simulink subsystem "atm"  (R2022b)
settings: Solver=VariableStepAuto  StartTime=0.0  StopTime=10.0  RelTol=1e-3
libraries: dspsigops x3
settings Model: Creator=padlewsk  LastModifiedBy=padlewsk

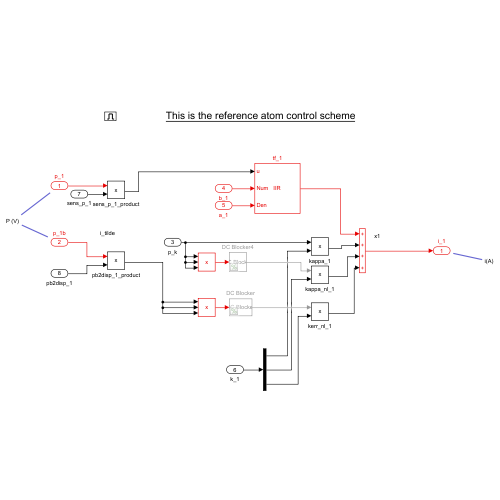
[thumbnail: Simulink's stored preview of the top-level diagram]
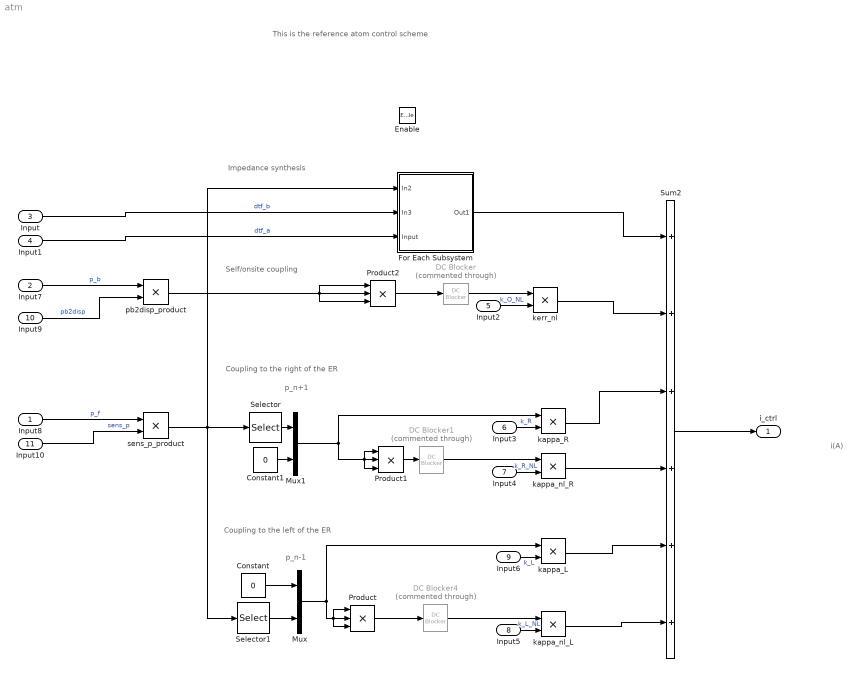
== system atm ==
  note: Impedance synthesis
  note: Coupling to the left of the ER
  note: Coupling to the right of the ER
  note: p_n-1
  note: This is the reference atom control scheme
  note: i(A)
  note: p_n+1
  note: Self/onsite coupling
  Input8 : Inport
  Input7 : Inport  Port=2
  Input : Inport  Port=3
  Input1 : Inport  Port=4
  Input2 : Inport  Port=5
  Input3 : Inport  Port=6
  Input4 : Inport  Port=7
  Input5 : Inport  Port=8
  Input6 : Inport  Port=9
  Input9 : Inport  Port=10
  Input10 : Inport  Port=11
  Enable : EnablePort
  Constant : Constant  Value=0
  Constant1 : Constant  Value=0
  DC Blocker : dspsigops/DC Blocker  Commented=through  Algorithm=FIR  NormalizedBandwidth=0.001  Length=50  Order=6  SimulateUsing=Code generation
      settings: LibrarySourceBlock=dsphdlsupportsigops/DC Blocker
  DC Blocker1 : dspsigops/DC Blocker  Commented=through  Algorithm=FIR  NormalizedBandwidth=0.001  Length=50  Order=6  SimulateUsing=Code generation
      settings: LibrarySourceBlock=dsphdlsupportsigops/DC Blocker
  DC Blocker4 : dspsigops/DC Blocker  Commented=through  Algorithm=FIR  NormalizedBandwidth=0.001  Length=50  Order=6  SimulateUsing=Code generation
      settings: LibrarySourceBlock=dsphdlsupportsigops/DC Blocker
  For Each Subsystem : Subsystem  TreatAsAtomicUnit=on
      settings: MinAlgLoopOccurrences=on  RTWSystemCode=Nonreusable function
  Mux : Mux  Inputs=2
  Mux1 : Mux  Inputs=2
  Product : Product  Inputs=3
  Product1 : Product  Inputs=3
  Product2 : Product  Inputs=3
  Selector : Selector  InputPortWidth=16  IndexOptions=Index vector (dialog)  Indices=[2:16]  OutputSizes=1
  Selector1 : Selector  InputPortWidth=16  IndexOptions=Index vector (dialog)  Indices=[1:15]  OutputSizes=1
  Sum2 : Sum  Inputs=++++++
  kappa_L : Product
  kappa_R : Product
  kappa_nl_L : Product
  kappa_nl_R : Product
  kerr_nl : Product
  pb2disp_product : Product
  sens_p_product : Product
  i_ctrl : Outport
  wires:
  Sum2/1 -> i_ctrl/1
  pb2disp_product/1 -> Product2/2, Product2/1, Product2/3
  Product/1 -> DC Blocker4/1
  DC Blocker4/1 -> kappa_nl_L/1
  DC Blocker/1 -> kerr_nl/1
  Product2/1 -> DC Blocker/1
  Product1/1 -> DC Blocker1/1
  DC Blocker1/1 -> kappa_nl_R/1
  kerr_nl/1 -> Sum2/2
  Constant/1 -> Mux/1
  Constant1/1 -> Mux1/2
  sens_p_product/1 -> Selector/1, Selector1/1, For Each Subsystem/1(In2)
  Mux1/1 -> Product1/2, Product1/1, Product1/3, kappa_R/1
  Mux/1 -> Product/2, Product/1, Product/3, kappa_L/1
  Selector/1 -> Mux1/1
  Selector1/1 -> Mux/2
  kappa_R/1 -> Sum2/3
  kappa_nl_R/1 -> Sum2/4
  kappa_L/1 -> Sum2/5
  kappa_nl_L/1 -> Sum2/6
  Input/1 -> For Each Subsystem/2(In3)  "dtf_b"
  Input1/1 -> For Each Subsystem/3(Input)  "dtf_a"
  Input4/1 -> kappa_nl_R/2  "k_R_NL"
  Input2/1 -> kerr_nl/2  "k_O_NL"
  Input3/1 -> kappa_R/2  "k_R"
  Input5/1 -> kappa_nl_L/2  "k_L_NL"
  Input6/1 -> kappa_L/2  "k_L"
  Input7/1 -> pb2disp_product/1  "p_b"
  Input8/1 -> sens_p_product/1  "p_f"
  Input9/1 -> pb2disp_product/2  "pb2disp"
  Input10/1 -> sens_p_product/2  "sens_p"
  For Each Subsystem/1(Out1) -> Sum2/1

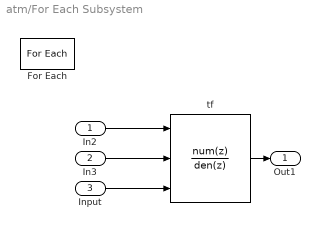
== system atm/For Each Subsystem ==
  In2 : Inport  Partition=on  PartitionDimension=1  PartitionWidth=1  PartitionOffset=0
  In3 : Inport  Port=2  Partition=on  PartitionDimension=1  PartitionWidth=1  PartitionOffset=0
  Input : Inport  Port=3  Partition=on  PartitionDimension=1  PartitionWidth=1  PartitionOffset=0
  For Each : ForEach  DisableCoverage=on
  tf : DiscreteTransferFcn  NumeratorSource=Input port  Numerator="[0.5         0.5         0.5]"  DenominatorSource=Input port  Denominator="[1  1  1]"  a0EqualsOne=on
      settings: InputPortMap=u0,p1,p3
  Out1 : Outport  ConcatenationDimension=1
  wires:
  Input/1 -> tf/3
  In3/1 -> tf/2
  tf/1 -> Out1/1
  In2/1 -> tf/1
